simulink model "onestdanslamerde"  (R2020a)
settings: Solver=VariableStepAuto  StartTime=0.0  StopTime=10.0  RelTol=1e-3
settings Model: Creator=lab02  LastModifiedBy=lab02

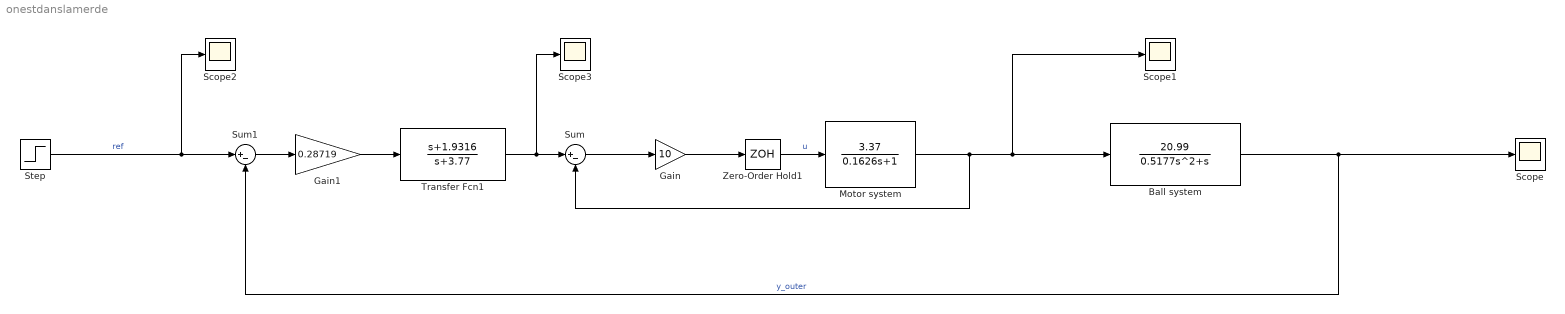
== system onestdanslamerde ==
  " Ball system" : TransferFcn  Numerator=[ 20.99]  Denominator=[0.5177 1 0]
  Gain : Gain  Gain=10
  Gain1 : Gain  Gain=0.28719
  Motor system : TransferFcn  Numerator=[0 3.37]  Denominator=[0.1626 1]
  Scope{,1..3} (4 alike) : Scope
  Step : Step
  Sum : Sum  Inputs=|+-
  Sum1 : Sum  Inputs=|+-
  Transfer Fcn1 : TransferFcn  Numerator=[1 1.9316]  Denominator=[1 3.77]
  Zero-Order Hold1 : ZeroOrderHold  SampleTime=0.005
  wires:
  Step/1 -> Sum1/1, Scope2/1  "ref"
  Gain1/1 -> Transfer Fcn1/1
  Transfer Fcn1/1 -> Sum/1, Scope3/1
  Sum1/1 -> Gain1/1
  " Ball system"/1 -> Sum1/2, Scope/1  "y_outer"
  Sum/1 -> Gain/1
  Zero-Order Hold1/1 -> Motor system/1  "u"
  Motor system/1 -> Sum/2, Scope1/1, " Ball system"/1
  Gain/1 -> Zero-Order Hold1/1
